simulink model "motor_starting_1"  (R2019b)
settings: Solver=ode23tb  StartTime=0.0  StopTime=60  RelTol=1e-3
undefined symbols (not defined in the file): D1, Delta
libraries: powerlib x13, powerlib_meascontrol x3
settings Model: Creator=a.abedi  LastModifiedBy=a.abedi

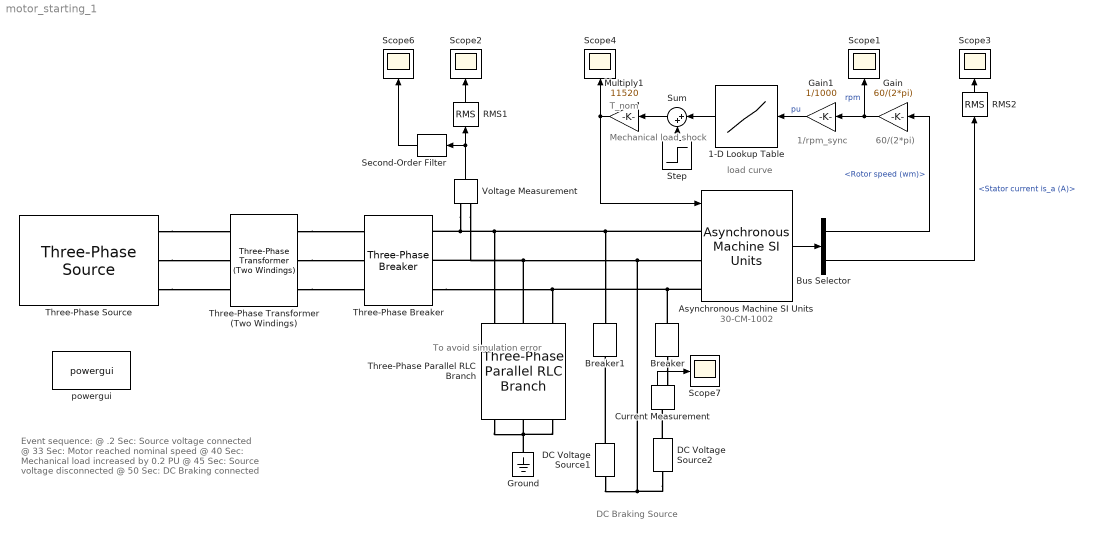
== system motor_starting_1 ==
  note: DC Braking Source
  note: To avoid
      | simulation
      | error
  note: Event sequence:
      | @ .2 Sec:	Source voltage connected
      | @ 33 Sec:	Motor reached nominal speed
      | @ 40 Sec:	Mechanical load increased by 0.2 PU
      | @ 45 Sec:	Source voltage disconnected
      | @ 50 Sec:	DC Braking connected
  note: Mechanical
      | load shock
  note: 30-CM-1002
  note: load curve
  note: T_nom
  note: 1/rpm_sync
  note: 60/(2*pi)
  1-D Lookup Table : Lookup_n-D  NumberOfTableDimensions=1  BreakpointsForDimension1=[0,1e-06,0.05,0.1,0.12,0.15,0.2,0.25,0.3,0.35,0.4,0.45,0.5,0.6,0.7,0.8,0.9,1,1.2,1.5,1.8,2.2]  Table=[0,0.07,0.035,0.012,0.011,0.012,0.017,0.025,0.034,0.049,0.061,0.079,0.097,0.14,0.187,0.245,0.305,0.375,0.54,0.8,1.1,1.5]  InternalRulePriority=Speed  RndMeth=Simplest  InputSameDT=on
  Asynchronous Machine SI Units : powerlib/Machines/Asynchronous Machine SI Units  RotorType=Double squirrel-cage  PresetModel=No  MechanicalLoad=Torque Tm  ShowDetailedParameters=on  ReferenceFrame=Rotor  Units=SI  MeasurementBus=off  NominalParameters=[1.2e+06 6000 50]  Stator=[0.6129 0.00968]  Rotor=[0.6258 0.005473]  Cage1=[0.1452 0.01024]  Cage2=[1.057 0.00968]  Lm=0.2818  Mechanical=[1844 30 3]  PolePairs=2  InitialConditions=[1 0 0 0 0 0 0 0]  SimulateSaturation=off  Saturation=[14.03593122, 27.81365428, 53.79336849, 72.68890987, 97.98006896, 148.6815601, 215.7428561, 302.9841135, 428.7778367 ; 230, 322, 414, 460, 506, 552, 598, 644, 690]  LoadFlowParameters=1492000  TsPowergui=0  TsBlock=-1  IterativeModel=Trapezoidal non iterative  IterativeDiscreteModel=Trapezoidal non iterative  Pmec=1.492e+006
      settings: SourceProductName=Simscape Electrical
  Breaker : powerlib/Elements/Breaker  InitialState=0  SwitchingTimes=[50]  External=off  BreakerResistance=0.01  SnubberResistance=1e6  SnubberCapacitance=inf  Measurements=None  MoreParameters=on  NoBreakLoop=off
      settings: SourceProductName=Simscape Electrical
  Breaker1 : powerlib/Elements/Breaker  InitialState=0  SwitchingTimes=[50]  External=off  BreakerResistance=0.01  SnubberResistance=1e6  SnubberCapacitance=inf  Measurements=None  MoreParameters=on  NoBreakLoop=off
      settings: SourceProductName=Simscape Electrical
  Bus Selector : BusSelector  OutputSignals=Mechanical.Rotor speed (wm),Stator measurements.Stator current is_a (A)
  Current Measurement : powerlib/Measurements/Current Measurement  PhasorSimulation=off  OutputType=Complex  PSBequivalent=0
      settings: SourceProductName=Simscape Electrical
  DC Voltage Source1 : powerlib/Electrical Sources/DC Voltage Source  Amplitude=1000  Measurements=None
      settings: SourceProductName=Simscape Electrical
  DC Voltage Source2 : powerlib/Electrical Sources/DC Voltage Source  Amplitude=1000  Measurements=None
      settings: SourceProductName=Simscape Electrical
  Gain : Gain  Gain=60/(2*pi)
  Gain1 : Gain  Gain=1/1000
  Ground : powerlib/Elements/Ground  LConnTagsString=a
      settings: SourceProductName=Simscape Electrical
  Multiply1 : Gain  Gain=11520
  RMS1 : powerlib_meascontrol/Measurements/RMS  TrueRMS=on  Freq=50  RMSInit=0  Ts=0
      settings: SourceProductName=Simscape Electrical
  RMS2 : powerlib_meascontrol/Measurements/RMS  TrueRMS=on  Freq=50  RMSInit=0  Ts=0
      settings: SourceProductName=Simscape Electrical
  Scope{1..4,6..7} (6 alike) : Scope
  Second-Order Filter : powerlib_meascontrol/Filters/Second-Order Filter  FilterType=Lowpass  Fo=100  Zeta=0.7  Ts=0  Initialize=on  Vac_Init="[0,  0,  50]"  Vdc_Init=0  PlotResponse=off  FreqRange=[0, 500, 1]
      settings: SourceProductName=Simscape Electrical  SourceProductBaseCode=PS
  Step : Step  Time=40  After=0.2  SampleTime=0
  Sum : Sum  Inputs=|++
  Three-Phase Parallel RLC Branch : powerlib/Elements/Three-Phase Parallel RLC Branch  LConnTagsString=A|B|C  RConnTagsString=A|B|C  BranchType=R  Resistance=1e3  Inductance=1e-3  Capacitance=0.1e-6  Measurements=None
      settings: SourceProductName=Simscape Electrical  SourceProductBaseCode=PS
  Three-Phase Transformer (Two Windings) : powerlib/Elements/Three-Phase Transformer (Two Windings)  Winding1Connection=Delta (D1)  Winding2Connection=Yg  CoreType=Three single-phase transformers  SetSaturation=off  Hysteresis=off  DataFile='hysteresis'  SetInitialFlux=off  Measurements=None  UNITS=pu  NominalPower=[ 20e6 , 50 ]  Winding1=[20e3 1e-3 0.04]  Winding2=[6.2e3 1e-3 0.04]  Rm=500  Lm=500  L0=0.5  Saturation=[0 0;0.0024001 1.2;0.99999 1.52]  InitialFluxes=[0.8 -0.8 0.7]  BreakLoop=off  DiscreteSolver=Trapezoidal iterative  DataType=off  TransfoNumber=1
      settings: SourceProductName=Simscape Electrical
  Three-Phase Breaker : powerlib/Elements/Three-Phase Breaker  InitialState=open  SwitchA=on  SwitchB=on  SwitchC=on  SwitchTimes=[0.2 45]  External=off  BreakerResistance=1e-6  SnubberResistance=1e6  SnubberCapacitance=inf  Measurements=None
      settings: SourceProductName=Simscape Electrical
  Three-Phase Source : powerlib/Electrical Sources/Three-Phase Source  InternalConnection=Yg  VoltagePhases=off  Voltage=20e3  PhaseAngle=0  Voltage_phases=[25e3 25e3 25e3]/sqrt(3)  PhaseAngles_phases=[0 -120 +120]  Frequency=50  NonIdealSource=on  SpecifyImpedance=on  Resistance=0.8929  Inductance=16.58e-3  ShortCircuitLevel=1000e6  BaseVoltage=20e3  XRratio=7  BusType=swing  Pref=10e3  Qref=0  Prefabc=[10e3, 10e3, 10e3]  Qrefabc=[0, 0, 0]  Qmin=-inf  Qmax=inf
      settings: SourceProductName=Simscape Electrical
  Voltage Measurement : powerlib/Measurements/Voltage Measurement  PhasorSimulation=off  OutputType=Magnitude  PSBequivalent=0
      settings: SourceProductName=Simscape Electrical
  powergui : powerlib/powergui  Priority=1  SimulationMode=Continuous  SampleTime=50e-6  frequency=50  Iterations=50  frequencyindice=50  Pbase=100e6  ErrMax=1e-4  UnitsV=kV  UnitsW=MW  buscounter=0  FunctionMessages=off  echomessages=off  EnableUseOfTLC=off  CurrentSourceSwitches=on  DisableSnubberDevices=off  DisableRonSwitches=off  DisableVfSwitches=off  DisplayEquations=off  AutomaticDiscreteSolvers=off  SolverType=Tustin/Backward Euler (TBE)  Interpol=off  ExternalGateDelay=off  methode=off  Ts=100  x0status=blocks  SPID=on  SwTol=0  HookPort=off  NonlinearTolerance=1e-4  nMaxIteration=100  ContinueOnMaxIteration=off  RestoreLinks=warning  ResistiveCurrentMeasurement=off  Frange=[0:2:500]  Ylog=off  Xlog=on  ShowGrid=off  save=off  variable=ZData  structure=0  ZoomFFT=off  StartTime=0.0  cycles=1  DisplayStyle=1  fundamental=60  FreqAxis=off  MaxFrequency=1000  frequencyindicesteady=1  RmsSteady=1  display=off
      settings: SourceProductName=Simscape Electrical
  wires:
  Bus Selector/2 -> RMS2/1  "<Stator current is_a (A)>"
  Bus Selector/1 -> Gain/1  "<Rotor speed (wm)>"
  Voltage Measurement/1 -> RMS1/1, Second-Order Filter/1
  RMS2/1 -> Scope3/1
  Asynchronous Machine SI Units/1 -> Bus Selector/1
  Gain/1 -> Scope1/1, Gain1/1  "rpm"
  Multiply1/1 -> Scope4/1, Asynchronous Machine SI Units/1
  RMS1/1 -> Scope2/1
  Gain1/1 -> 1-D Lookup Table/1  "pu"
  1-D Lookup Table/1 -> Sum/1
  Sum/1 -> Multiply1/1
  Step/1 -> Sum/2
  Second-Order Filter/1 -> Scope6/1
  Current Measurement/1 -> Scope7/1
  connections:
  Three-Phase Transformer (Two Windings)/RConn3 -- Three-Phase Breaker/LConn3
  Three-Phase Transformer (Two Windings)/RConn2 -- Three-Phase Breaker/LConn2
  Three-Phase Transformer (Two Windings)/RConn1 -- Three-Phase Breaker/LConn1
  Three-Phase Source/RConn3 -- Three-Phase Transformer (Two Windings)/LConn3
  Three-Phase Source/RConn2 -- Three-Phase Transformer (Two Windings)/LConn2
  Three-Phase Source/RConn1 -- Three-Phase Transformer (Two Windings)/LConn1
  Asynchronous Machine SI Units/LConn3 -- Three-Phase Breaker/RConn3 -- Three-Phase Parallel RLC Branch/LConn3 -- Breaker/RConn1
  Asynchronous Machine SI Units/LConn1 -- Breaker1/RConn1 -- Three-Phase Breaker/RConn1 -- Voltage Measurement/LConn1 -- Three-Phase Parallel RLC Branch/LConn1
  Ground/LConn1 -- Three-Phase Parallel RLC Branch/RConn3 -- Three-Phase Parallel RLC Branch/RConn1 -- Three-Phase Parallel RLC Branch/RConn2
  DC Voltage Source1/LConn1 -- DC Voltage Source2/LConn1 -- Voltage Measurement/LConn2 -- Three-Phase Breaker/RConn2 -- Three-Phase Parallel RLC Branch/LConn2 -- Asynchronous Machine SI Units/LConn2
  DC Voltage Source1/RConn1 -- Breaker1/LConn1
  DC Voltage Source2/RConn1 -- Current Measurement/LConn1
  Breaker/LConn1 -- Current Measurement/RConn1
